simulink model "simulation_poursuite_discret"  (Simulink 7.6)
settings: Solver=ode45  StartTime=0  StopTime=15  RelTol=1e-3
values from neighbouring files (symbols this model uses):
  den_IMC = [1 -1]    [syntheseReg.m]
  num_IMC = 3.70429313276254e-005*[1 1]    [syntheseReg.m]
  Te = 0.00001    (= 1e-05)    [syntheseReg.m]
libraries: simulink x1, cstblocks x1
settings Model: Creator=Nicolas  LastModifiedBy=Igor

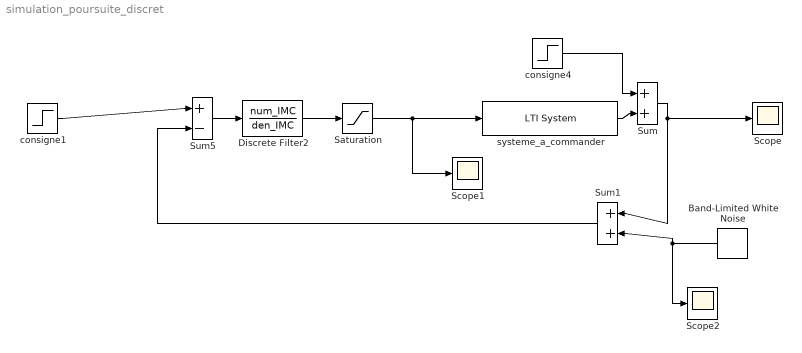
== system simulation_poursuite_discret ==
  Band-Limited White Noise : simulink/Sources/Band-Limited White Noise  SystemSampleTime=-1  Cov=[0.0000001]  Ts=Te  seed=[23341]
  Discrete Filter2 : DiscreteFilter  Numerator=num_IMC  Denominator=den_IMC  SampleTime=Te
  Saturation : Saturate  UpperLimit=0.8  LowerLimit=0  SampleTime=Te
  Scope : Scope
      settings: TimeRange=1.5  YMin=-9.999999999999999e+305  YMax=3.5e+306  MaxDataPoints=50000  SampleInput=on  SampleTime=Te
  Scope1 : Scope
      settings: TimeRange=5  YMin=0.1  YMax=1  MaxDataPoints=50000  SampleInput=on  SampleTime=Te
  Scope2 : Scope
      settings: TimeRange=1.5  YMin=-9.999999999999999e+305  YMax=3.5e+306  SaveName=ScopeData2  MaxDataPoints=50000  SampleInput=on  SampleTime=Te
  Sum : Sum  Inputs=|++  SampleTime=Te
  Sum1 : Sum  Inputs=|++  SampleTime=Te
  Sum5 : Sum  Inputs=|+-  SampleTime=Te
  consigne1 : Step  After=36  SampleTime=Te
  consigne4 : Step  Time=5  SampleTime=Te
  systeme_a_commander : cstblocks/LTI System  SystemSampleTime=-1  sys=G_disc4  IC=[]
  wires:
  Sum5/1 -> Discrete Filter2/1
  systeme_a_commander/1 -> Sum/2
  Sum/1 -> Scope/1, Sum1/1
  Discrete Filter2/1 -> Saturation/1
  Saturation/1 -> Scope1/1, systeme_a_commander/1
  consigne1/1 -> Sum5/1
  consigne4/1 -> Sum/1
  Sum1/1 -> Sum5/2
  Band-Limited White Noise/1 -> Sum1/2, Scope2/1
